simulink model "ThdRwStOccupyChk_logic"  (R2018b)
settings: Solver=VariableStepAuto  StartTime=0.0  StopTime=10.0  RelTol=1e-3
undefined symbols (not defined in the file or in its folder): SeatOccupiedSts1
libraries: Lib x3
settings Model: Creator=sn2xws  LastModifiedBy=sn2xws

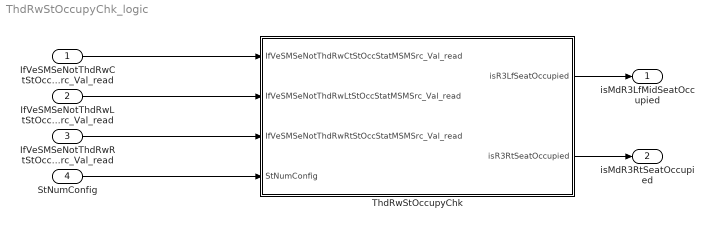
== system ThdRwStOccupyChk_logic ==
  IfVeSMSeNotThdRwCtStOccStatMSMSrc_Val_read : Inport
  IfVeSMSeNotThdRwLtStOccStatMSMSrc_Val_read : Inport  Port=2
  IfVeSMSeNotThdRwRtStOccStatMSMSrc_Val_read : Inport  Port=3
  StNumConfig : Inport  Port=4
  ThdRwStOccupyChk : Subsystem
  isMdR3LfMidSeatOccupied : Outport
  isMdR3RtSeatOccupied : Outport  Port=2
  wires:
  IfVeSMSeNotThdRwLtStOccStatMSMSrc_Val_read/1 -> ThdRwStOccupyChk/2(IfVeSMSeNotThdRwLtStOccStatMSMSrc_Val_read)
  StNumConfig/1 -> ThdRwStOccupyChk/4(StNumConfig)
  IfVeSMSeNotThdRwCtStOccStatMSMSrc_Val_read/1 -> ThdRwStOccupyChk/1(IfVeSMSeNotThdRwCtStOccStatMSMSrc_Val_read)
  ThdRwStOccupyChk/2(isR3RtSeatOccupied) -> isMdR3RtSeatOccupied/1
  IfVeSMSeNotThdRwRtStOccStatMSMSrc_Val_read/1 -> ThdRwStOccupyChk/3(IfVeSMSeNotThdRwRtStOccStatMSMSrc_Val_read)
  ThdRwStOccupyChk/1(isR3LfSeatOccupied) -> isMdR3LfMidSeatOccupied/1

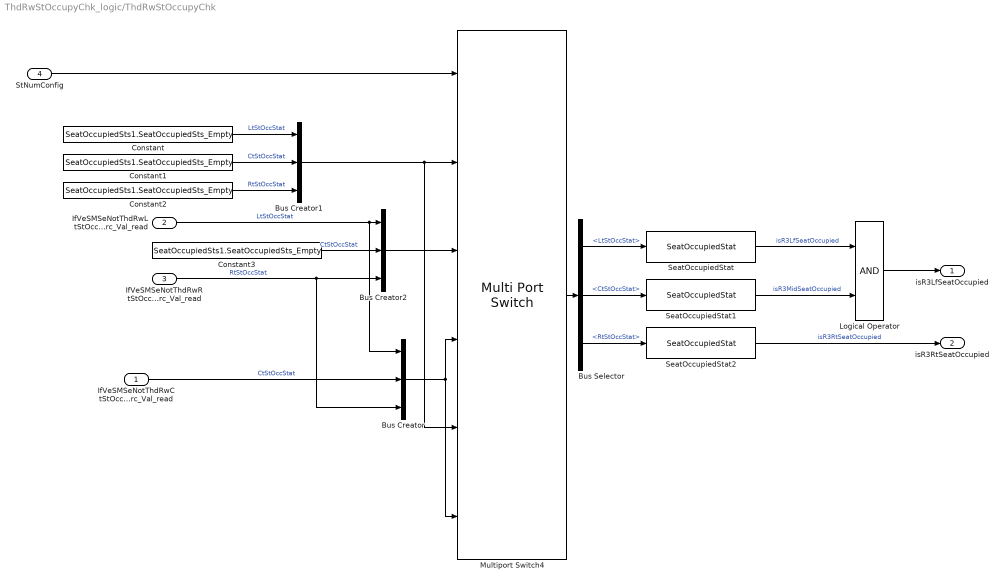
== system ThdRwStOccupyChk_logic/ThdRwStOccupyChk ==
  IfVeSMSeNotThdRwCtStOccStatMSMSrc_Val_read : Inport
  IfVeSMSeNotThdRwLtStOccStatMSMSrc_Val_read : Inport  Port=2
  IfVeSMSeNotThdRwRtStOccStatMSMSrc_Val_read : Inport  Port=3
  StNumConfig : Inport  Port=4
  Bus Creator : BusCreator  Inputs=3
  Bus Creator1 : BusCreator  Inputs=3
  Bus Creator2 : BusCreator  Inputs=3
  Bus Selector : BusSelector  OutputSignals=LtStOccStat,CtStOccStat,RtStOccStat
  Constant{,1..3} (4 alike) : Constant  Value=SeatOccupiedSts1.SeatOccupiedSts_Empty  OutDataTypeStr=Enum:SeatOccupiedSts1
  Logical Operator : Logic  AllPortsSameDT=off  OutDataTypeStr=boolean
  Multiport Switch4 : MultiPortSwitch  DataPortOrder=Specify indices  DataPortIndices={IfVeSMSeStNumConfig.SeatNum4Config,IfVeSMSeStNumConfig.SeatNum6Config,IfVeSMSeStNumConfig.SeatNum7Config,IfVeSMSeStNumConfig.SeatNum4PConfig}  DataPortForDefault=Additional data port  DiagnosticForDefault=None
  SeatOccupiedStat : Lib/SeatOccupiedStat  SystemSampleTime=-1
  SeatOccupiedStat1 : Lib/SeatOccupiedStat  SystemSampleTime=-1
  SeatOccupiedStat2 : Lib/SeatOccupiedStat  SystemSampleTime=-1
  isR3LfSeatOccupied : Outport
  isR3RtSeatOccupied : Outport  Port=2
  wires:
  SeatOccupiedStat/1 -> Logical Operator/1  "isR3LfSeatOccupied"
  SeatOccupiedStat2/1 -> isR3RtSeatOccupied/1  "isR3RtSeatOccupied"
  StNumConfig/1 -> Multiport Switch4/1
  IfVeSMSeNotThdRwCtStOccStatMSMSrc_Val_read/1 -> Bus Creator/2  "CtStOccStat"
  Bus Creator/1 -> Multiport Switch4/6, Multiport Switch4/4
  Multiport Switch4/1 -> Bus Selector/1
  Constant2/1 -> Bus Creator1/3  "RtStOccStat"
  Constant/1 -> Bus Creator1/1  "LtStOccStat"
  Bus Creator1/1 -> Multiport Switch4/2, Multiport Switch4/5
  Constant1/1 -> Bus Creator1/2  "CtStOccStat"
  Constant3/1 -> Bus Creator2/2  "CtStOccStat"
  Bus Creator2/1 -> Multiport Switch4/3
  IfVeSMSeNotThdRwLtStOccStatMSMSrc_Val_read/1 -> Bus Creator/1, Bus Creator2/1  "LtStOccStat"
  IfVeSMSeNotThdRwRtStOccStatMSMSrc_Val_read/1 -> Bus Creator2/3, Bus Creator/3  "RtStOccStat"
  Bus Selector/1 -> SeatOccupiedStat/1  "<LtStOccStat>"
  Bus Selector/2 -> SeatOccupiedStat1/1  "<CtStOccStat>"
  Bus Selector/3 -> SeatOccupiedStat2/1  "<RtStOccStat>"
  SeatOccupiedStat1/1 -> Logical Operator/2  "isR3MidSeatOccupied"
  Logical Operator/1 -> isR3LfSeatOccupied/1
